simulink model "mrefrobotarm_modified_previous_y_previous_u_previous_ref_pert_2"  (R2018b)
settings: Solver=FixedStepAuto  StartTime=0.0  StopTime=60  RelTol=1e-3  AbsTol=1e-6
undefined symbols (not defined in the file or in its folder): cc, options
libraries: neural x858, simulink x1
(part 6 of 32)

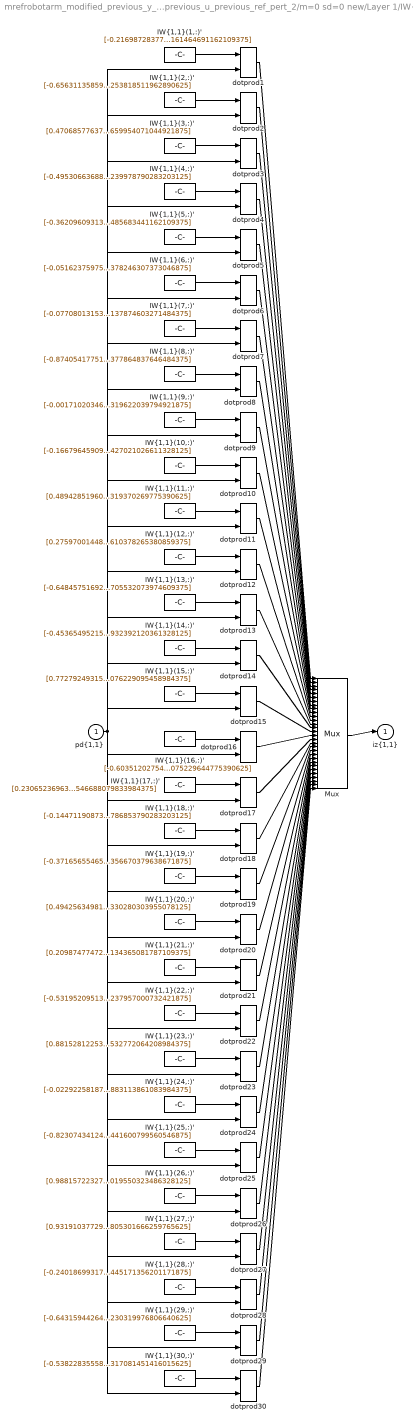
== system mrefrobotarm_modified_previous_y_previous_u_previous_ref_pert_2/m=0 sd=0 new/Layer 1/IW{1,1} ==
  "pd{1,1}" : Inport  PortDimensions=10
      mask Display: e = 0.06;c1 = [120 230 180]/255;c2 = ([120 230 180]+0)/(256+128);c3 = ([120 230 180]+128)/(256+128);patch([0 1 1 0],[0 0 1 1],c1);patch([0 1 1 1-e 1-e 0+e],[0 0 1 1-e 0+e 0+e],c2);patch([0 0 1 1-e 0+e 0+e],[0 1 1 1-e 1-e 0+e],c3);plot([0 1 1 0 0],[0 0 1 1 0]);
  "IW{1,1}(1,:)'" : Constant  Value=[-0.216987283771066963300455654461984522640705108642578125;0.62705080224373699326889664007467217743396759033203125;-0.8295293486517885117592641108785755932331085205078125;0.393994151975692596945322065948857925832271575927734375;0.62619892286198453046353051831829361617565155029296875;0.8292962339521758874383294823928736150264739990234375;-1.098156613770668865726065632770769298076629638671875;0.2506190603631857083399836483295075595378875732421875;0.50722615998603115539111740872613154351711273193359375;0.1507590943215458556547758917076862417161464691162109375]
      mask Display: e = 0.06;c1 = [120 150 230]/255;c2 = ([120 150 230]+0)/383;c3 = ([120 150 230]+128)/383;patch([0 1 1 0],[0 0 1 1],c1);patch([0 1 1 1-e 1-e 0+e],[0 0 1 1-e 0+e 0+e],c2);patch([0 0 1 1-e 0+e 0+e],[0 1 1 1-e 1-e 0+e],c3);plot([0 1 1 0 0],[0 0 1 1 0]);disp('Weights');
  "IW{1,1}(10,:)'" : Constant  Value=[-0.16679645909830032035614522101241163909435272216796875;-0.6842996916674486396203747062827460467815399169921875;-0.630369694434009364414350784500129520893096923828125;0.730752341665734217457384147564880549907684326171875;0.4034951403199287245371351673384197056293487548828125;0.00078084238114074062085678828992740818648599088191986083984375;0.7993574007866841579783567794947884976863861083984375;0.609031860504884559048832670669071376323699951171875;-0.63394148118544768610860273838625289499759674072265625;0.272956076386066559535947817494161427021026611328125]
      mask Display: e = 0.06;c1 = [120 150 230]/255;c2 = ([120 150 230]+0)/383;c3 = ([120 150 230]+128)/383;patch([0 1 1 0],[0 0 1 1],c1);patch([0 1 1 1-e 1-e 0+e],[0 0 1 1-e 0+e 0+e],c2);patch([0 0 1 1-e 0+e 0+e],[0 1 1 1-e 1-e 0+e],c3);plot([0 1 1 0 0],[0 0 1 1 0]);disp('Weights');
  "IW{1,1}(11,:)'" : Constant  Value=[0.489428519601812050954237065525376237928867340087890625;-0.7365528190820691545326326377107761800289154052734375;-0.451546779372395568064035842326120473444461822509765625;0.1405859040881517196819316950495704077184200286865234375;-0.93048882369243612888709549224586226046085357666015625;-0.26211444689542295893858181443647481501102447509765625;0.08561728287347047938737887307070195674896240234375;0.55048760249225259233440965545014478266239166259765625;0.9806074606537305005105054078740067780017852783203125;0.79905409092773960200162264300161041319370269775390625]
      mask Display: e = 0.06;c1 = [120 150 230]/255;c2 = ([120 150 230]+0)/383;c3 = ([120 150 230]+128)/383;patch([0 1 1 0],[0 0 1 1],c1);patch([0 1 1 1-e 1-e 0+e],[0 0 1 1-e 0+e 0+e],c2);patch([0 0 1 1-e 0+e 0+e],[0 1 1 1-e 1-e 0+e],c3);plot([0 1 1 0 0],[0 0 1 1 0]);disp('Weights');
  "IW{1,1}(12,:)'" : Constant  Value=[0.2759700144846828351319345529191195964813232421875;-0.71241257184170303506931531956070102751255035400390625;0.75486500134028045039258358883671462535858154296875;0.381454650786102245074715710870805196464061737060546875;0.004858777844072236472283687902518067858181893825531005859375;0.6166915534499739504070703333127312362194061279296875;-0.3196849222814306390461069895536638796329498291015625;0.002620030545543486875936789459728970541618764400482177734375;0.473104586099457879999619080990669317543506622314453125;0.5512413222707603921435293159447610378265380859375]
      mask Display: e = 0.06;c1 = [120 150 230]/255;c2 = ([120 150 230]+0)/383;c3 = ([120 150 230]+128)/383;patch([0 1 1 0],[0 0 1 1],c1);patch([0 1 1 1-e 1-e 0+e],[0 0 1 1-e 0+e 0+e],c2);patch([0 0 1 1-e 0+e 0+e],[0 1 1 1-e 1-e 0+e],c3);plot([0 1 1 0 0],[0 0 1 1 0]);disp('Weights');
  "IW{1,1}(13,:)'" : Constant  Value=[-0.6484575169221555857035355074913240969181060791015625;-0.499724694266350244475916042574681341648101806640625;0.495700138337080653538890828713192604482173919677734375;0.34971064326349843298658015555702149868011474609375;-0.060241231962616825779122109452146105468273162841796875;0.8259595789221894079901176155544817447662353515625;-0.1282548551957359561637161959879449568688869476318359375;0.367966930034267447613416379681439138948917388916015625;0.475561097872065297043064902027253992855548858642578125;0.70652399157070566726446259053773246705532073974609375]
      mask Display: e = 0.06;c1 = [120 150 230]/255;c2 = ([120 150 230]+0)/383;c3 = ([120 150 230]+128)/383;patch([0 1 1 0],[0 0 1 1],c1);patch([0 1 1 1-e 1-e 0+e],[0 0 1 1-e 0+e 0+e],c2);patch([0 0 1 1-e 0+e 0+e],[0 1 1 1-e 1-e 0+e],c3);plot([0 1 1 0 0],[0 0 1 1 0]);disp('Weights');
  "IW{1,1}(14,:)'" : Constant  Value=[-0.453654952159654012433520620106719434261322021484375;-0.087078018426318681832754009519703686237335205078125;1.2183161916568605587229967568418942391872406005859375;0.188480531629046710317965107606141828000545501708984375;0.1578055972773705073475269955451949499547481536865234375;0.5630549301229657022105357100372202694416046142578125;-0.478321804103466641233666223342879675328731536865234375;-0.64260437295462813356294873301521874964237213134765625;-0.65210239962574600980360628454945981502532958984375;-0.40497145512570142944497320058871991932392120361328125]
      mask Display: e = 0.06;c1 = [120 150 230]/255;c2 = ([120 150 230]+0)/383;c3 = ([120 150 230]+128)/383;patch([0 1 1 0],[0 0 1 1],c1);patch([0 1 1 1-e 1-e 0+e],[0 0 1 1-e 0+e 0+e],c2);patch([0 0 1 1-e 0+e 0+e],[0 1 1 1-e 1-e 0+e],c3);plot([0 1 1 0 0],[0 0 1 1 0]);disp('Weights');
  "IW{1,1}(15,:)'" : Constant  Value=[0.7727924931534893016049636571551673114299774169921875;0.60406524780855430645232218012097291648387908935546875;-0.339234357772328964930608208305784501135349273681640625;-0.3665639941056635375815631050500087440013885498046875;-0.556871153861037360144337071687914431095123291015625;0.644694140791529424205918985535390675067901611328125;-0.223918537202554890352956817878293804824352264404296875;0.3929628245523184570942021309747360646724700927734375;0.02724513081364417221852392003711429424583911895751953125;0.81554675643314966659858100683777593076229095458984375]
      mask Display: e = 0.06;c1 = [120 150 230]/255;c2 = ([120 150 230]+0)/383;c3 = ([120 150 230]+128)/383;patch([0 1 1 0],[0 0 1 1],c1);patch([0 1 1 1-e 1-e 0+e],[0 0 1 1-e 0+e 0+e],c2);patch([0 0 1 1-e 0+e 0+e],[0 1 1 1-e 1-e 0+e],c3);plot([0 1 1 0 0],[0 0 1 1 0]);disp('Weights');
  "IW{1,1}(16,:)'" : Constant  Value=[-0.6035120275440231107921817965689115226268768310546875;0.2650624083125163732432838514796458184719085693359375;0.1664063050611622462948702150242752395570278167724609375;-0.604589080027903236214115167967975139617919921875;0.90825794261307823962425800345954485237598419189453125;-0.47690630518536381021732495355536229908466339111328125;-0.35494856231991367412348381549236364662647247314453125;0.466535944338989594371014391072094440460205078125;-0.780215681548742878703706082887947559356689453125;-0.3376554549046739683859641445451416075229644775390625]
      mask Display: e = 0.06;c1 = [120 150 230]/255;c2 = ([120 150 230]+0)/383;c3 = ([120 150 230]+128)/383;patch([0 1 1 0],[0 0 1 1],c1);patch([0 1 1 1-e 1-e 0+e],[0 0 1 1-e 0+e 0+e],c2);patch([0 0 1 1-e 0+e 0+e],[0 1 1 1-e 1-e 0+e],c3);plot([0 1 1 0 0],[0 0 1 1 0]);disp('Weights');
  "IW{1,1}(17,:)'" : Constant  Value=[0.2306523696345013363373510628662188537418842315673828125;-0.66846711145320103497624586452730000019073486328125;-0.41967272211457673503076648557907901704311370849609375;-0.091567790243069768774120120724546723067760467529296875;-0.398592563146790868078284120201715268194675445556640625;-0.279877438869719608049990711151622235774993896484375;0.82883291633788058749843230543774552643299102783203125;-0.1333171916388301847522512844079756177961826324462890625;-0.6301658819520257193147472207783721387386322021484375;0.5355902885660466239414745359681546688079833984375]
      mask Display: e = 0.06;c1 = [120 150 230]/255;c2 = ([120 150 230]+0)/383;c3 = ([120 150 230]+128)/383;patch([0 1 1 0],[0 0 1 1],c1);patch([0 1 1 1-e 1-e 0+e],[0 0 1 1-e 0+e 0+e],c2);patch([0 0 1 1-e 0+e 0+e],[0 1 1 1-e 1-e 0+e],c3);plot([0 1 1 0 0],[0 0 1 1 0]);disp('Weights');
  "IW{1,1}(18,:)'" : Constant  Value=[-0.1447119087393781977635143221050384454429149627685546875;-0.67475381623391406105127998671378009021282196044921875;0.4926578834720551913761710238759405910968780517578125;0.70749694307740629284353417460806667804718017578125;-0.81313721438408492758753709495067596435546875;-0.6308535590054675790128158041625283658504486083984375;1.066570045903236785278522802400402724742889404296875;-0.1087662439031829297864106820270535536110401153564453125;0.09858723671447215675112119015466305427253246307373046875;0.9426396597433364110685261039179749786853790283203125]
      mask Display: e = 0.06;c1 = [120 150 230]/255;c2 = ([120 150 230]+0)/383;c3 = ([120 150 230]+128)/383;patch([0 1 1 0],[0 0 1 1],c1);patch([0 1 1 1-e 1-e 0+e],[0 0 1 1-e 0+e 0+e],c2);patch([0 0 1 1-e 0+e 0+e],[0 1 1 1-e 1-e 0+e],c3);plot([0 1 1 0 0],[0 0 1 1 0]);disp('Weights');
  "IW{1,1}(19,:)'" : Constant  Value=[-0.371656554659357152292642467728001065552234649658203125;-0.7018845097005816935364919118001125752925872802734375;1.0316394152161632025155313385766930878162384033203125;0.5557190202728887751248976201168261468410491943359375;-0.1863534602959450448000922051505767740309238433837890625;-0.72915117971346810055166542952065356075763702392578125;0.91600930480328390803634874828276224434375762939453125;0.1577223946696830469971217780766892246901988983154296875;0.85902723150752902103732822070014663040637969970703125;0.64534881990236925286552605030010454356670379638671875]
      mask Display: e = 0.06;c1 = [120 150 230]/255;c2 = ([120 150 230]+0)/383;c3 = ([120 150 230]+128)/383;patch([0 1 1 0],[0 0 1 1],c1);patch([0 1 1 1-e 1-e 0+e],[0 0 1 1-e 0+e 0+e],c2);patch([0 0 1 1-e 0+e 0+e],[0 1 1 1-e 1-e 0+e],c3);plot([0 1 1 0 0],[0 0 1 1 0]);disp('Weights');
  "IW{1,1}(2,:)'" : Constant  Value=[-0.656311358597397198622047653771005570888519287109375;0.6210564788165158223165462914039380848407745361328125;0.94659452939866473020202874977258034050464630126953125;0.341720850421762867288322240710840560495853424072265625;0.52399770718595373164561124212923459708690643310546875;-0.11255994669816392350636391483931220136582851409912109375;-0.629474985561337074813081926549784839153289794921875;0.54818420872382522812671368228620849549770355224609375;0.382682863478270018919857875516754575073719024658203125;-0.358137010837502212101668419563793577253818511962890625]
      mask Display: e = 0.06;c1 = [120 150 230]/255;c2 = ([120 150 230]+0)/383;c3 = ([120 150 230]+128)/383;patch([0 1 1 0],[0 0 1 1],c1);patch([0 1 1 1-e 1-e 0+e],[0 0 1 1-e 0+e 0+e],c2);patch([0 0 1 1-e 0+e 0+e],[0 1 1 1-e 1-e 0+e],c3);plot([0 1 1 0 0],[0 0 1 1 0]);disp('Weights');
  "IW{1,1}(20,:)'" : Constant  Value=[0.494256349816460716084520754520781338214874267578125;0.6449621240293150759015361472847871482372283935546875;-0.548925345535696163068450914579443633556365966796875;0.1607665954672680419523800310344086028635501861572265625;0.5095365243905012331282478044158779084682464599609375;-0.46606007941572025199405970852239988744258880615234375;0.7077983047368852087544155438081361353397369384765625;0.1819713578390899366699073880226933397352695465087890625;-0.58909671703797716890704805337009020149707794189453125;0.41197545162792881257018962060101330280303955078125]
      mask Display: e = 0.06;c1 = [120 150 230]/255;c2 = ([120 150 230]+0)/383;c3 = ([120 150 230]+128)/383;patch([0 1 1 0],[0 0 1 1],c1);patch([0 1 1 1-e 1-e 0+e],[0 0 1 1-e 0+e 0+e],c2);patch([0 0 1 1-e 0+e 0+e],[0 1 1 1-e 1-e 0+e],c3);plot([0 1 1 0 0],[0 0 1 1 0]);disp('Weights');
  "IW{1,1}(21,:)'" : Constant  Value=[0.2098747747229458837647797508907387964427471160888671875;-0.5831388250806190942654438913450576364994049072265625;-0.8125065083100049267983422396355308592319488525390625;-0.1640580210739865929525649335118941962718963623046875;0.1851608194018606601272125544710434041917324066162109375;-0.87381318513758443611294524089316837489604949951171875;-0.6439644679846081576357619269401766359806060791015625;0.849195408431800746740236718324013054370880126953125;-0.70272659898133926770213975032675080001354217529296875;0.2487594358167200814246911022564745508134365081787109375]
      mask Display: e = 0.06;c1 = [120 150 230]/255;c2 = ([120 150 230]+0)/383;c3 = ([120 150 230]+128)/383;patch([0 1 1 0],[0 0 1 1],c1);patch([0 1 1 1-e 1-e 0+e],[0 0 1 1-e 0+e 0+e],c2);patch([0 0 1 1-e 0+e 0+e],[0 1 1 1-e 1-e 0+e],c3);plot([0 1 1 0 0],[0 0 1 1 0]);disp('Weights');
  "IW{1,1}(22,:)'" : Constant  Value=[-0.53195209513385022237486055018962360918521881103515625;0.6519075330133146106703634359291754662990570068359375;-0.00984206405327076212785630815460535814054310321807861328125;0.2282313297764917425780595294781960546970367431640625;0.5819370594691435361056619512964971363544464111328125;-0.96429911237563625814317447293433360755443572998046875;0.49354997350437501690834096734761260449886322021484375;-0.1671444002196741662746859446997405029833316802978515625;0.32939011148036534404326403091545216739177703857421875;-0.377391799678823580688202810051734559237957000732421875]
      mask Display: e = 0.06;c1 = [120 150 230]/255;c2 = ([120 150 230]+0)/383;c3 = ([120 150 230]+128)/383;patch([0 1 1 0],[0 0 1 1],c1);patch([0 1 1 1-e 1-e 0+e],[0 0 1 1-e 0+e 0+e],c2);patch([0 0 1 1-e 0+e 0+e],[0 1 1 1-e 1-e 0+e],c3);plot([0 1 1 0 0],[0 0 1 1 0]);disp('Weights');
  "IW{1,1}(23,:)'" : Constant  Value=[0.8815281225349613780650770422653295099735260009765625;0.40270018845487276504258034037775360047817230224609375;0.57991893310328845867474001352093182504177093505859375;-0.5129980514669953972628491101204417645931243896484375;-0.223966997186081540061053374301991425454616546630859375;-0.366294231918401269609830706031061708927154541015625;-0.06265200727221575949243970171664841473102569580078125;-0.61398951057415829257735140345175750553607940673828125;-0.30705887589114488900321475739474408328533172607421875;0.190830137831930757297271838979213498532772064208984375]
      mask Display: e = 0.06;c1 = [120 150 230]/255;c2 = ([120 150 230]+0)/383;c3 = ([120 150 230]+128)/383;patch([0 1 1 0],[0 0 1 1],c1);patch([0 1 1 1-e 1-e 0+e],[0 0 1 1-e 0+e 0+e],c2);patch([0 0 1 1-e 0+e 0+e],[0 1 1 1-e 1-e 0+e],c3);plot([0 1 1 0 0],[0 0 1 1 0]);disp('Weights');
  "IW{1,1}(24,:)'" : Constant  Value=[-0.0229225818708987984229086265486330376006662845611572265625;-0.7364519044524120428008018279797397553920745849609375;0.36430817379126245736387090801144950091838836669921875;0.5435151814966214800506350002251565456390380859375;0.5390086111008420832746423911885358393192291259765625;-0.404702945706581107554455911667901091277599334716796875;-0.060098154716755392001914515276439487934112548828125;-0.5263787975544593766841217075125314295291900634765625;-0.63371890806124342443439445560215972363948822021484375;-0.530579493924592693332442649989388883113861083984375]
      mask Display: e = 0.06;c1 = [120 150 230]/255;c2 = ([120 150 230]+0)/383;c3 = ([120 150 230]+128)/383;patch([0 1 1 0],[0 0 1 1],c1);patch([0 1 1 1-e 1-e 0+e],[0 0 1 1-e 0+e 0+e],c2);patch([0 0 1 1-e 0+e 0+e],[0 1 1 1-e 1-e 0+e],c3);plot([0 1 1 0 0],[0 0 1 1 0]);disp('Weights');
  "IW{1,1}(25,:)'" : Constant  Value=[-0.8230743412482983689670845706132240593433380126953125;-0.0272604362854576599828337890585316927172243595123291015625;0.64641548903671408599080905332812108099460601806640625;-0.0203134078178269193715177465264787315391004085540771484375;-0.258650719593879252489188047547941096127033233642578125;-0.62706624270569566448330078856088221073150634765625;0.0243146746468201717383816884421321447007358074188232421875;-0.52779963376747074388362079844227991998195648193359375;0.1553783024495765108241585039650090038776397705078125;-0.76378718712697757364793460510554723441600799560546875]
      mask Display: e = 0.06;c1 = [120 150 230]/255;c2 = ([120 150 230]+0)/383;c3 = ([120 150 230]+128)/383;patch([0 1 1 0],[0 0 1 1],c1);patch([0 1 1 1-e 1-e 0+e],[0 0 1 1-e 0+e 0+e],c2);patch([0 0 1 1-e 0+e 0+e],[0 1 1 1-e 1-e 0+e],c3);plot([0 1 1 0 0],[0 0 1 1 0]);disp('Weights');
  "IW{1,1}(26,:)'" : Constant  Value=[0.98815722327362054411281633292674086987972259521484375;0.0552131657533536379656169401641818694770336151123046875;-0.418257496746552270838748199821566231548786163330078125;-0.05024649133487103791484429393676691688597202301025390625;-0.80753775333930766233692111200070939958095550537109375;0.08673093154260026749202694418272585608065128326416015625;0.92391389942989643468962412953260354697704315185546875;0.1278291914222002556567048259239527396857738494873046875;0.1560718371625417211223663116470561362802982330322265625;0.77398147285488960722688034366001375019550323486328125]
      mask Display: e = 0.06;c1 = [120 150 230]/255;c2 = ([120 150 230]+0)/383;c3 = ([120 150 230]+128)/383;patch([0 1 1 0],[0 0 1 1],c1);patch([0 1 1 1-e 1-e 0+e],[0 0 1 1-e 0+e 0+e],c2);patch([0 0 1 1-e 0+e 0+e],[0 1 1 1-e 1-e 0+e],c3);plot([0 1 1 0 0],[0 0 1 1 0]);disp('Weights');
  "IW{1,1}(27,:)'" : Constant  Value=[0.93191037729317127702444167880457825958728790283203125;0.60668600265606309474009094628854654729366302490234375;-0.777303014667443559204684788710437715053558349609375;-0.08537723853186175715368477767697186209261417388916015625;0.130164040371312073052223468039301224052906036376953125;0.28580205238479938767426347112632356584072113037109375;0.373812544658363332672479373286478221416473388671875;-0.1759004421836329046247016094639548100531101226806640625;-0.094785177444393908796627101764897815883159637451171875;0.6758158633839619344740867745713330805301666259765625]
      mask Display: e = 0.06;c1 = [120 150 230]/255;c2 = ([120 150 230]+0)/383;c3 = ([120 150 230]+128)/383;patch([0 1 1 0],[0 0 1 1],c1);patch([0 1 1 1-e 1-e 0+e],[0 0 1 1-e 0+e 0+e],c2);patch([0 0 1 1-e 0+e 0+e],[0 1 1 1-e 1-e 0+e],c3);plot([0 1 1 0 0],[0 0 1 1 0]);disp('Weights');
  "IW{1,1}(28,:)'" : Constant  Value=[-0.2401869931725169327041413680490222759544849395751953125;0.0933490469089056362772538477656780742108821868896484375;0.283965118888948431230545565995271317660808563232421875;-0.375273050517266393288906556335859932005405426025390625;0.06775152256870629885465717734405188821256160736083984375;-0.2128280154068902529918005939180147834122180938720703125;0.7029462040397820299375553076970390975475311279296875;-0.18189905831341868225337066178326494991779327392578125;-0.88707246082706003864615240672719664871692657470703125;-1.365924164345173164036850721458904445171356201171875]
      mask Display: e = 0.06;c1 = [120 150 230]/255;c2 = ([120 150 230]+0)/383;c3 = ([120 150 230]+128)/383;patch([0 1 1 0],[0 0 1 1],c1);patch([0 1 1 1-e 1-e 0+e],[0 0 1 1-e 0+e 0+e],c2);patch([0 0 1 1-e 0+e 0+e],[0 1 1 1-e 1-e 0+e],c3);plot([0 1 1 0 0],[0 0 1 1 0]);disp('Weights');
  "IW{1,1}(29,:)'" : Constant  Value=[-0.64315944264548396969161103697842918336391448974609375;0.6524413609077208686670701354159973561763763427734375;0.13025818837213420930964957733522169291973114013671875;-0.67229574107036016439309378256439231336116790771484375;-0.84247495097735447533437991296523250639438629150390625;-0.32742522553510211569260945907444693148136138916015625;0.69578690917679353322711222062935121357440948486328125;0.051313881836411778802897742934874258935451507568359375;0.64190761578990918057030512500205077230930328369140625;0.43682643035762058758564307936467230319976806640625]
      mask Display: e = 0.06;c1 = [120 150 230]/255;c2 = ([120 150 230]+0)/383;c3 = ([120 150 230]+128)/383;patch([0 1 1 0],[0 0 1 1],c1);patch([0 1 1 1-e 1-e 0+e],[0 0 1 1-e 0+e 0+e],c2);patch([0 0 1 1-e 0+e 0+e],[0 1 1 1-e 1-e 0+e],c3);plot([0 1 1 0 0],[0 0 1 1 0]);disp('Weights');
  "IW{1,1}(3,:)'" : Constant  Value=[0.47068577637060970975113605163642205297946929931640625;-0.81747315534249043178505189644056372344493865966796875;0.45053305837691037805115001901867799460887908935546875;-0.0548758257766226720253399662396986968815326690673828125;-0.1605704134370416202859388477008906193077564239501953125;1.2029143395823604922867389177554287016391754150390625;-0.81216427835985982586208820066531188786029815673828125;-0.01570430564939097328736039571595028974115848541259765625;0.414564087612156628726012286279001273214817047119140625;0.794648975814773006476343653048388659954071044921875]
      mask Display: e = 0.06;c1 = [120 150 230]/255;c2 = ([120 150 230]+0)/383;c3 = ([120 150 230]+128)/383;patch([0 1 1 0],[0 0 1 1],c1);patch([0 1 1 1-e 1-e 0+e],[0 0 1 1-e 0+e 0+e],c2);patch([0 0 1 1-e 0+e 0+e],[0 1 1 1-e 1-e 0+e],c3);plot([0 1 1 0 0],[0 0 1 1 0]);disp('Weights');
  "IW{1,1}(30,:)'" : Constant  Value=[-0.53822835558789605681084822208504192531108856201171875;1.159787663619848974150272624683566391468048095703125;-0.86501236586838070596883198959403671324253082275390625;-0.1231851979617612780071311817664536647498607635498046875;-0.51277279413427756526999701236491091549396514892578125;0.689416509994279724793386776582337915897369384765625;-0.42621795881081758761155242609675042331218719482421875;0.048422457052984792247318779345732764340937137603759765625;-0.131929430229489330628211973817087709903717041015625;0.48884396801740681581804892630316317081451416015625]
      mask Display: e = 0.06;c1 = [120 150 230]/255;c2 = ([120 150 230]+0)/383;c3 = ([120 150 230]+128)/383;patch([0 1 1 0],[0 0 1 1],c1);patch([0 1 1 1-e 1-e 0+e],[0 0 1 1-e 0+e 0+e],c2);patch([0 0 1 1-e 0+e 0+e],[0 1 1 1-e 1-e 0+e],c3);plot([0 1 1 0 0],[0 0 1 1 0]);disp('Weights');
  "IW{1,1}(4,:)'" : Constant  Value=[-0.49530663688463760774283173304866068065166473388671875;0.6136403433405799301425531666609458625316619873046875;0.85233958134315745969189492825535126030445098876953125;0.165792313211370168080094344986719079315662384033203125;0.56325187075390459323642744493554346263408660888671875;0.277628373818218865398677053235587663948535919189453125;-0.42389833454236247600732667706324718892574310302734375;-0.20937666051480963158581971583771519362926483154296875;1.0465057893284377410481056358548812568187713623046875;0.1900015937802159993186279507426661439239978790283203125]
      mask Display: e = 0.06;c1 = [120 150 230]/255;c2 = ([120 150 230]+0)/383;c3 = ([120 150 230]+128)/383;patch([0 1 1 0],[0 0 1 1],c1);patch([0 1 1 1-e 1-e 0+e],[0 0 1 1-e 0+e 0+e],c2);patch([0 0 1 1-e 0+e 0+e],[0 1 1 1-e 1-e 0+e],c3);plot([0 1 1 0 0],[0 0 1 1 0]);disp('Weights');
  "IW{1,1}(5,:)'" : Constant  Value=[-0.3620960931350583056342884447076357901096343994140625;1.130102095756748692423343527480028569698333740234375;-0.7039825232618814876417445702827535569667816162109375;0.046549796347439449661909094402290065772831439971923828125;0.5881263061220682875074317053076811134815216064453125;-1.0852232563820314314995130189345218241214752197265625;0.56574130436339753469354718617978505790233612060546875;0.1653429641065014277234723749643308110535144805908203125;-0.60252530532840176125120024153147824108600616455078125;-0.52934170901582111579131151302135549485683441162109375]
      mask Display: e = 0.06;c1 = [120 150 230]/255;c2 = ([120 150 230]+0)/383;c3 = ([120 150 230]+128)/383;patch([0 1 1 0],[0 0 1 1],c1);patch([0 1 1 1-e 1-e 0+e],[0 0 1 1-e 0+e 0+e],c2);patch([0 0 1 1-e 0+e 0+e],[0 1 1 1-e 1-e 0+e],c3);plot([0 1 1 0 0],[0 0 1 1 0]);disp('Weights');
  "IW{1,1}(6,:)'" : Constant  Value=[-0.0516237597593852959310112282764748670160770416259765625;-0.245458975940660961700956477216095663607120513916015625;0.53802875658127125024776660211500711739063262939453125;0.3693960386380628069247222811100073158740997314453125;1.060992725645990564231624375679530203342437744140625;0.55496448811041443338609724378329701721668243408203125;-0.60147789323544176287583695739158429205417633056640625;-0.27984504580453284372509870081557892262935638427734375;0.5428421998752817057010133794392459094524383544921875;-0.3295573414571772996595200311276130378246307373046875]
      mask Display: e = 0.06;c1 = [120 150 230]/255;c2 = ([120 150 230]+0)/383;c3 = ([120 150 230]+128)/383;patch([0 1 1 0],[0 0 1 1],c1);patch([0 1 1 1-e 1-e 0+e],[0 0 1 1-e 0+e 0+e],c2);patch([0 0 1 1-e 0+e 0+e],[0 1 1 1-e 1-e 0+e],c3);plot([0 1 1 0 0],[0 0 1 1 0]);disp('Weights');
  "IW{1,1}(7,:)'" : Constant  Value=[-0.07708013153856636823224590671088662929832935333251953125;-0.87590647446304092937907626037485897541046142578125;0.58717235701994019425598025918588973581790924072265625;0.5962857812360355946879053590237163007259368896484375;-0.1590429756890310020178702643534052185714244842529296875;-0.509116171235311387732735965983010828495025634765625;0.86633314081629386738114817489986307919025421142578125;0.290534077645184130034294867073185741901397705078125;-0.27408168723662218457803874116507358849048614501953125;-0.6646354326505858889362343688844703137874603271484375]
      mask Display: e = 0.06;c1 = [120 150 230]/255;c2 = ([120 150 230]+0)/383;c3 = ([120 150 230]+128)/383;patch([0 1 1 0],[0 0 1 1],c1);patch([0 1 1 1-e 1-e 0+e],[0 0 1 1-e 0+e 0+e],c2);patch([0 0 1 1-e 0+e 0+e],[0 1 1 1-e 1-e 0+e],c3);plot([0 1 1 0 0],[0 0 1 1 0]);disp('Weights');
  "IW{1,1}(8,:)'" : Constant  Value=[-0.87405417751009439886189511526026763021945953369140625;-0.346756480088971696940092215299955569207668304443359375;0.34684900409427787959515399052179418504238128662109375;-0.708096296216499165865343456971459090709686279296875;0.07833996096102800732463578015085658989846706390380859375;0.007723425516580014783818430856854320154525339603424072265625;-0.54297909870956673206165987721760757267475128173828125;0.0738216637421419130671296215950860641896724700927734375;-0.70374845398028529341871717406320385634899139404296875;-0.1048515085895514731273436837000190280377864837646484375]
      mask Display: e = 0.06;c1 = [120 150 230]/255;c2 = ([120 150 230]+0)/383;c3 = ([120 150 230]+128)/383;patch([0 1 1 0],[0 0 1 1],c1);patch([0 1 1 1-e 1-e 0+e],[0 0 1 1-e 0+e 0+e],c2);patch([0 0 1 1-e 0+e 0+e],[0 1 1 1-e 1-e 0+e],c3);plot([0 1 1 0 0],[0 0 1 1 0]);disp('Weights');
  "IW{1,1}(9,:)'" : Constant  Value=[-0.0017102034643802256630440439266749308444559574127197265625;0.4539323608377834329274946867371909320354461669921875;-0.806122733135806956994429128826595842838287353515625;0.3381836592315432543642828022711910307407379150390625;-1.07107356088941241267775694723241031169891357421875;0.2282814433906463491563698653408209793269634246826171875;1.123741852508879812688746824278496205806732177734375;-0.31979190850257743772289131811703555285930633544921875;-0.46961328404062019359344049007631838321685791015625;0.049962947523143057260153199194974149577319622039794921875]
      mask Display: e = 0.06;c1 = [120 150 230]/255;c2 = ([120 150 230]+0)/383;c3 = ([120 150 230]+128)/383;patch([0 1 1 0],[0 0 1 1],c1);patch([0 1 1 1-e 1-e 0+e],[0 0 1 1-e 0+e 0+e],c2);patch([0 0 1 1-e 0+e 0+e],[0 1 1 1-e 1-e 0+e],c3);plot([0 1 1 0 0],[0 0 1 1 0]);disp('Weights');
  Mux : Mux  Inputs=30
      mask Display: e = 0.06;c1 = [120 150 230]/255;c2 = ([120 150 230]+0)/383;c3 = ([120 150 230]+128)/383;patch([0 1 1 0],[0 0 1 1],c1);patch([0 1 1 1-e 1-e 0+e],[0 0 1 1-e 0+e 0+e],c2);patch([0 0 1 1-e 0+e 0+e],[0 1 1 1-e 1-e 0+e],c3);plot([0 1 1 0 0],[0 0 1 1 0]);disp('Mux');
  dotprod{1..30} (30 alike) : neural/Weight Functions/dotprod
  "iz{1,1}" : Outport
      mask Display: e = 0.06;c1 = [120 230 180]/255;c2 = ([120 230 180]+0)/(256+128);c3 = ([120 230 180]+128)/(256+128);patch([0 1 1 0],[0 0 1 1],c1);patch([0 1 1 1-e 1-e 0+e],[0 0 1 1-e 0+e 0+e],c2);patch([0 0 1 1-e 0+e 0+e],[0 1 1 1-e 1-e 0+e],c3);plot([0 1 1 0 0],[0 0 1 1 0]);
  wires:
  "IW{1,1}(1,:)'"/1 -> dotprod1/1
  "pd{1,1}"/1 -> dotprod1/2, dotprod2/2, dotprod3/2, dotprod4/2, dotprod5/2, dotprod6/2, dotprod7/2, dotprod8/2, dotprod9/2, dotprod10/2, dotprod11/2, dotprod12/2, dotprod13/2, dotprod14/2, dotprod15/2, dotprod16/2, dotprod17/2, dotprod18/2, dotprod19/2, dotprod20/2, dotprod21/2, dotprod22/2, dotprod23/2, dotprod24/2, dotprod25/2, dotprod26/2, dotprod27/2, dotprod28/2, dotprod29/2, dotprod30/2
  dotprod1/1 -> Mux/1
  "IW{1,1}(2,:)'"/1 -> dotprod2/1
  dotprod2/1 -> Mux/2
  "IW{1,1}(3,:)'"/1 -> dotprod3/1
  dotprod3/1 -> Mux/3
  "IW{1,1}(4,:)'"/1 -> dotprod4/1
  dotprod4/1 -> Mux/4
  "IW{1,1}(5,:)'"/1 -> dotprod5/1
  dotprod5/1 -> Mux/5
  "IW{1,1}(6,:)'"/1 -> dotprod6/1
  dotprod6/1 -> Mux/6
  "IW{1,1}(7,:)'"/1 -> dotprod7/1
  dotprod7/1 -> Mux/7
  "IW{1,1}(8,:)'"/1 -> dotprod8/1
  dotprod8/1 -> Mux/8
  "IW{1,1}(9,:)'"/1 -> dotprod9/1
  dotprod9/1 -> Mux/9
  "IW{1,1}(10,:)'"/1 -> dotprod10/1
  dotprod10/1 -> Mux/10
  "IW{1,1}(11,:)'"/1 -> dotprod11/1
  dotprod11/1 -> Mux/11
  "IW{1,1}(12,:)'"/1 -> dotprod12/1
  dotprod12/1 -> Mux/12
  "IW{1,1}(13,:)'"/1 -> dotprod13/1
  dotprod13/1 -> Mux/13
  "IW{1,1}(14,:)'"/1 -> dotprod14/1
  dotprod14/1 -> Mux/14
  "IW{1,1}(15,:)'"/1 -> dotprod15/1
  dotprod15/1 -> Mux/15
  "IW{1,1}(16,:)'"/1 -> dotprod16/1
  dotprod16/1 -> Mux/16
  "IW{1,1}(17,:)'"/1 -> dotprod17/1
  dotprod17/1 -> Mux/17
  "IW{1,1}(18,:)'"/1 -> dotprod18/1
  dotprod18/1 -> Mux/18
  "IW{1,1}(19,:)'"/1 -> dotprod19/1
  dotprod19/1 -> Mux/19
  "IW{1,1}(20,:)'"/1 -> dotprod20/1
  dotprod20/1 -> Mux/20
  "IW{1,1}(21,:)'"/1 -> dotprod21/1
  dotprod21/1 -> Mux/21
  "IW{1,1}(22,:)'"/1 -> dotprod22/1
  dotprod22/1 -> Mux/22
  "IW{1,1}(23,:)'"/1 -> dotprod23/1
  dotprod23/1 -> Mux/23
  "IW{1,1}(24,:)'"/1 -> dotprod24/1
  dotprod24/1 -> Mux/24
  "IW{1,1}(25,:)'"/1 -> dotprod25/1
  dotprod25/1 -> Mux/25
  "IW{1,1}(26,:)'"/1 -> dotprod26/1
  dotprod26/1 -> Mux/26
  "IW{1,1}(27,:)'"/1 -> dotprod27/1
  dotprod27/1 -> Mux/27
  "IW{1,1}(28,:)'"/1 -> dotprod28/1
  dotprod28/1 -> Mux/28
  "IW{1,1}(29,:)'"/1 -> dotprod29/1
  dotprod29/1 -> Mux/29
  "IW{1,1}(30,:)'"/1 -> dotprod30/1
  dotprod30/1 -> Mux/30
  Mux/1 -> "iz{1,1}"/1

== system mrefrobotarm_modified_previous_y_previous_u_previous_ref_pert_2/m=0 sd=0 new/Layer 2/Delays 1 ==
  "p{2}" : Inport  PortDimensions=30
      mask Display: e = 0.06;c1 = [120 230 180]/255;c2 = ([120 230 180]+0)/(256+128);c3 = ([120 230 180]+128)/(256+128);patch([0 1 1 0],[0 0 1 1],c1);patch([0 1 1 1-e 1-e 0+e],[0 0 1 1-e 0+e 0+e],c2);patch([0 0 1 1-e 0+e 0+e],[0 1 1 1-e 1-e 0+e],c3);plot([0 1 1 0 0],[0 0 1 1 0]);
  mux : Mux  Inputs=1
      mask Display: e = 0.06;c1 = [120 150 230]/255;c2 = ([120 150 230]+0)/383;c3 = ([120 150 230]+128)/383;patch([0 1 1 0],[0 0 1 1],c1);patch([0 1 1 1-e 1-e 0+e],[0 0 1 1-e 0+e 0+e],c2);patch([0 0 1 1-e 0+e 0+e],[0 1 1 1-e 1-e 0+e],c3);plot([0 1 1 0 0],[0 0 1 1 0]);disp('Mux')
  "pd{2,1}" : Outport
      mask Display: e = 0.06;c1 = [120 230 180]/255;c2 = ([120 230 180]+0)/(256+128);c3 = ([120 230 180]+128)/(256+128);patch([0 1 1 0],[0 0 1 1],c1);patch([0 1 1 1-e 1-e 0+e],[0 0 1 1-e 0+e 0+e],c2);patch([0 0 1 1-e 0+e 0+e],[0 1 1 1-e 1-e 0+e],c3);plot([0 1 1 0 0],[0 0 1 1 0]);
  wires:
  "p{2}"/1 -> mux/1
  mux/1 -> "pd{2,1}"/1
